simulink model "foward"  (R2021a)
settings: Solver=VariableStepAuto  StartTime=0.0  StopTime=10.0  RelTol=1e-3
settings Model: Creator=abdul  LastModifiedBy=abdul

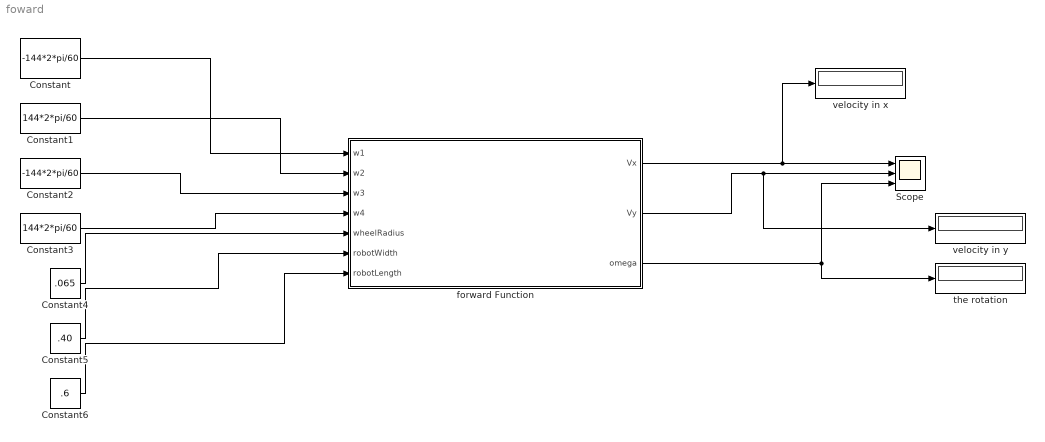
== system foward ==
  Constant : Constant  Value=-144*2*pi/60
  Constant1 : Constant  Value=144*2*pi/60
  Constant2 : Constant  Value=-144*2*pi/60
  Constant3 : Constant  Value=144*2*pi/60
  Constant4 : Constant  Value=.065
  Constant5 : Constant  Value=.40
  Constant6 : Constant  Value=.6
  Scope : Scope  NumInputPorts=3
  forward Function : MATLAB Function  TreatAsAtomicUnit=on
  the rotation : Display
  velocity in x : Display
  velocity in y : Display
  wires:
  Constant/1 -> forward Function/1(w1)
  Constant1/1 -> forward Function/2(w2)
  Constant2/1 -> forward Function/3(w3)
  Constant3/1 -> forward Function/4(w4)
  Constant4/1 -> forward Function/5(wheelRadius)
  Constant5/1 -> forward Function/6(robotWidth)
  Constant6/1 -> forward Function/7(robotLength)
  forward Function/1(Vx) -> velocity in x/1, Scope/1
  forward Function/2(Vy) -> velocity in y/1, Scope/2
  forward Function/3(omega) -> Scope/3, the rotation/1

== matlab function foward/forward Function ==
  data: w1 input; Vx output; w2 input; w3 input; w4 input; wheelRadius input; robotWidth input; robotLength input; Vy output; omega output
function [Vx, Vy, omega] = mecanumForwardKinematics(w1, w2, w3, w4, wheelRadius, robotWidth, robotLength)
    % Forward Kinematics for Mecanum Wheeled Robot
    R = wheelRadius;
    L = robotWidth / 2;
    d = robotLength / 2;
    o=L+d;

    M = [
         1   ,1   ,1    , 1 ;
        -1   ,1   ,1    ,-1 ;
        -1/o ,1/o ,-1/o ,1/o; 
    ];

    W = [w1; w2; w3; w4];
    X_dot = R/4.*M * W;

    Vx = X_dot(1);
    Vy = X_dot(2);
    omega = X_dot(3);
end
